simulink model "MON_sl_after_replacement3"  (R2016a)
settings: Solver=FixedStepDiscrete  StartTime=0.0  StopTime=10.0  RelTol=1e-3
undefined symbols (not defined in the file or in its folder): BRAKE_PRESSURE_LO, BRAKE_PRESSURE_MAX, BRAKE_PRESSURE_MED, dt, LO, MANUAL, MAX, MED
libraries: BSCU_lib x3, simulink x1
Description:
  | BSCU Monitor Function Model
settings Model: ModelType=Feature  MBDTemplateVer=1.1  sldv_blockreplacement_configurable_lib=MON_sl_after_rt3_lib  LastModifiedBy=jdbackes
settings DataIOCC: LimitDataPoints=on
settings DebuggingCC: ArtificialAlgebraicLoopMsg=none  AllowSymbolicDim=off
settings ModelReferenceCC: PropagateSignalLabelsOutOfModel=off
settings RTWCC: Description=Generic Real-Time Target
settings GRTTargetCC: GeneratePreprocessorConditionals=Use local settings
settings ConfigComp: DVMode=PropertyProving  DVTestSuiteOptimization=CombinedObjectives (Nonlinear Extended)  DVAssertions=EnableAll  DVProofAssumptions=EnableAll  DVDisplayReport=off

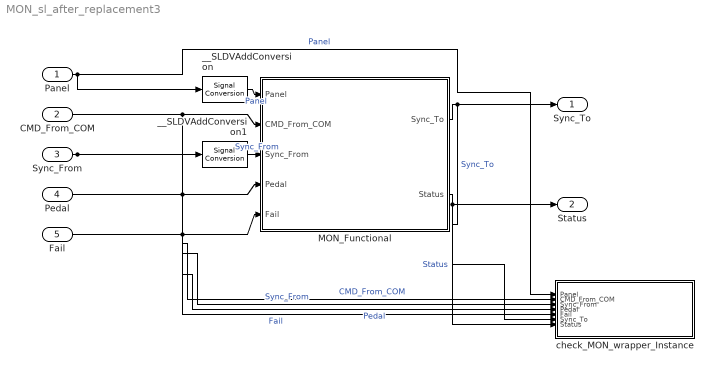
== system MON_sl_after_replacement3 ==
  Panel : Inport  OutDataTypeStr=Bus: PanelMsgImpl  SampleTime=dt  Interpolate=off  BusOutputAsStruct=on
  CMD_From_COM : Inport  Port=2  OutDataTypeStr=int32  SampleTime=dt  Interpolate=off
  Sync_From : Inport  Port=3  OutDataTypeStr=Bus: SyncMsgImpl  SampleTime=dt  Interpolate=off  BusOutputAsStruct=on
  Pedal : Inport  Port=4  OutDataTypeStr=int32  SampleTime=dt  Interpolate=off
  Fail : Inport  Port=5  OutDataTypeStr=boolean  SampleTime=dt  Interpolate=off
  MON_Functional : Subsystem  TreatAsAtomicUnit=on  mask(Sldv ModelReference(Model name:MON_Functional) Replacement){ModelName=MON_Functional, ParameterArgumentNames=, ParameterArgumentValues=, SimulationMode=Normal}
      mask help: Replacement for the Model Reference block that references the model MON_Functional. If Model arguments are specified on the Model Reference block, then they will appear in the mask parameters.
  __SLDVAddConversion : SignalConversion  ConversionOutput=Virtual bus  OverrideOpt=off
  __SLDVAddConversion1 : SignalConversion  ConversionOutput=Virtual bus  OverrideOpt=off
  check_MON_wrapper_Instance : MATLAB Function  TreatAsAtomicUnit=on  mask(VerificationSubsystem){}
  Sync_To : Outport  OutDataTypeStr=Bus: SyncMsgImpl  BusOutputAsStruct=on
  Status : Outport  Port=2  OutDataTypeStr=Bus: ChannelStatusImpl  BusOutputAsStruct=on
  wires:
  MON_Functional/1(Sync_To) -> Sync_To/1, check_MON_wrapper_Instance/6(Sync_To)  "Sync_To"
  MON_Functional/2(Status) -> Status/1, check_MON_wrapper_Instance/7(Status)  "Status"
  Panel/1 -> check_MON_wrapper_Instance/1(Panel), __SLDVAddConversion/1  "Panel"
  CMD_From_COM/1 -> MON_Functional/2(CMD_From_COM), check_MON_wrapper_Instance/2(CMD_From_COM)  "CMD_From_COM"
  Sync_From/1 -> check_MON_wrapper_Instance/3(Sync_From), __SLDVAddConversion1/1  "Sync_From"
  Pedal/1 -> MON_Functional/4(Pedal), check_MON_wrapper_Instance/4(Pedal)  "Pedal"
  Fail/1 -> MON_Functional/5(Fail), check_MON_wrapper_Instance/5(Fail)  "Fail"
  __SLDVAddConversion/1 -> MON_Functional/1(Panel)  "Panel"
  __SLDVAddConversion1/1 -> MON_Functional/3(Sync_From)  "Sync_From"

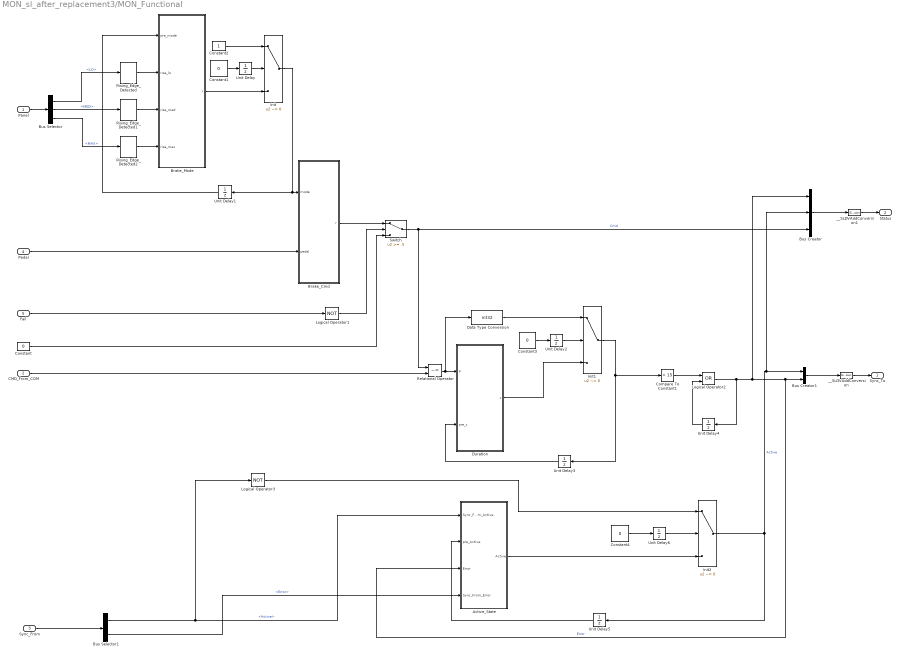
== system MON_sl_after_replacement3/MON_Functional ==
  Panel : Inport  OutDataTypeStr=Bus: PanelMsgImpl  SampleTime=[0.01,0]
  CMD_From_COM : Inport  Port=2  OutDataTypeStr=int32  PortDimensions=1  SampleTime=[0.01,0]
  Sync_From : Inport  Port=3  OutDataTypeStr=Bus: SyncMsgImpl  SampleTime=[0.01,0]
  Pedal : Inport  Port=4  OutDataTypeStr=int32  PortDimensions=1  SampleTime=[0.01,0]
  Fail : Inport  Port=5  OutDataTypeStr=boolean  PortDimensions=1  SampleTime=[0.01,0]
  Active_State : Stateflow chart  TreatAsAtomicUnit=on
  Brake_Cmd : Stateflow chart  TreatAsAtomicUnit=on
  Brake_Mode : Stateflow chart  TreatAsAtomicUnit=on
  Bus Creator : BusCreator  Inputs='Error','Active','Cmd'  OutDataTypeStr=Bus: ChannelStatusImpl  NonVirtualBus=on
  Bus Creator1 : BusCreator  Inputs='Active','Error'  OutDataTypeStr=Bus: SyncMsgImpl  NonVirtualBus=on
  Bus Selector : BusSelector  OutputSignals=LO,MED,MAX
  Bus Selector1 : BusSelector  OutputSignals=Active,Error
  Compare To Constant1 : simulink/Logic and Bit Operations/Compare To Constant  relop=>  const=15  OutDataTypeStr=boolean
  Constant : Constant  Value=0  OutDataTypeStr=int32
  Constant1 : Constant  DisableCoverage=on  Value=0  OutDataTypeStr=boolean
  Constant2 : Constant  OutDataTypeStr=int32
  Constant3 : Constant  DisableCoverage=on  Value=0  OutDataTypeStr=boolean
  Constant4 : Constant  DisableCoverage=on  Value=0  OutDataTypeStr=boolean
  Data Type Conversion : DataTypeConversion  OutDataTypeStr=int32
  Duration : Stateflow chart  TreatAsAtomicUnit=on
  Init : Switch  Criteria=u2 ~= 0  OutDataTypeStr=Inherit: Inherit via back propagation  ZeroCross=off  InputSameDT=on
  Init1 : Switch  Criteria=u2 ~= 0  OutDataTypeStr=Inherit: Inherit via back propagation  ZeroCross=off  InputSameDT=on
  Init2 : Switch  Criteria=u2 ~= 0  OutDataTypeStr=Inherit: Inherit via back propagation  ZeroCross=off  InputSameDT=on
  Logical Operator1 : Logic  Operator=NOT  OutDataTypeStr=boolean
  Logical Operator2 : Logic  Operator=OR  OutDataTypeStr=boolean
  Logical Operator3 : Logic  Operator=NOT  OutDataTypeStr=boolean
  Relational Operator : RelationalOperator  Operator=~=  OutDataTypeStr=boolean  ZeroCross=off  InputSameDT=on
  Rising_Edge_Detected : BSCU_lib/Rising_Edge_Detected
  Rising_Edge_Detected1 : BSCU_lib/Rising_Edge_Detected
  Rising_Edge_Detected2 : BSCU_lib/Rising_Edge_Detected
  Switch : Switch  Description=May be used within well defined functions, or functions that soley define logical expressions.  Threshold=.5  ZeroCross=off  InputSameDT=on
  Unit Delay{,1..2,6} (4 alike) : UnitDelay  InitialCondition=1  SampleTime=-1
      settings: AttributesFormatString=<Init = %<InitialCondition>>
  Unit Delay3 : UnitDelay  SampleTime=-1
      settings: AttributesFormatString=<Init = %<InitialCondition>>
  Unit Delay4 : UnitDelay  SampleTime=-1
      settings: AttributesFormatString=<Init = %<InitialCondition>>
  Unit Delay5 : UnitDelay  SampleTime=-1
      settings: AttributesFormatString=<Init = %<InitialCondition>>
  __SLDVAddConversion : SignalConversion  ConversionOutput=Virtual bus  OverrideOpt=off
  __SLDVAddConversion1 : SignalConversion  ConversionOutput=Virtual bus  OverrideOpt=off
  Sync_To : Outport  OutDataTypeStr=Bus: SyncMsgImpl
  Status : Outport  Port=2  OutDataTypeStr=Bus: ChannelStatusImpl
  wires:
  Unit Delay6/1 -> Init2/2
  Unit Delay5/1 -> Active_State/2(pre_Active)
  Unit Delay4/1 -> Logical Operator2/2
  Unit Delay3/1 -> Duration/2(pre_c)
  Unit Delay1/1 -> Brake_Mode/1(pre_mode)
  Init2/1 -> Unit Delay5/1, Bus Creator/2, Bus Creator1/1  "Active"
  Logical Operator3/1 -> Init2/1
  Constant4/1 -> Unit Delay6/1
  Active_State/1(Active) -> Init2/3
  Init1/1 -> Compare To Constant1/1, Unit Delay3/1
  Data Type Conversion/1 -> Init1/1
  Constant3/1 -> Unit Delay2/1
  Unit Delay2/1 -> Init1/2
  Duration/1(c) -> Init1/3
  Constant2/1 -> Init/1
  Constant1/1 -> Unit Delay/1
  Unit Delay/1 -> Init/2
  Bus Selector1/2 -> Active_State/4(Sync_From_Error)  "<Error>"
  Bus Selector1/1 -> Logical Operator3/1, Active_State/1(Sync_From_Active)  "<Active>"
  Sync_From/1 -> Bus Selector1/1
  Compare To Constant1/1 -> Logical Operator2/1
  Logical Operator2/1 -> Unit Delay4/1, Bus Creator/1, Active_State/3(Error), Bus Creator1/2  "Error"
  Relational Operator/1 -> Data Type Conversion/1, Duration/1(p)
  CMD_From_COM/1 -> Relational Operator/2
  Constant/1 -> Switch/3
  Switch/1 -> Bus Creator/3, Relational Operator/1  "Cmd"
  Logical Operator1/1 -> Switch/2
  Brake_Cmd/1(r) -> Switch/1
  Fail/1 -> Logical Operator1/1
  Pedal/1 -> Brake_Cmd/2(pedal)
  Rising_Edge_Detected2/1 -> Brake_Mode/4(rise_max)
  Rising_Edge_Detected1/1 -> Brake_Mode/3(rise_med)
  Rising_Edge_Detected/1 -> Brake_Mode/2(rise_lo)
  Bus Selector/3 -> Rising_Edge_Detected2/1  "<MAX>"
  Bus Selector/2 -> Rising_Edge_Detected1/1  "<MED>"
  Bus Selector/1 -> Rising_Edge_Detected/1  "<LO>"
  Panel/1 -> Bus Selector/1
  Init/1 -> Unit Delay1/1, Brake_Cmd/1(mode)
  Brake_Mode/1(r) -> Init/3
  Bus Creator1/1 -> __SLDVAddConversion/1
  __SLDVAddConversion/1 -> Sync_To/1
  Bus Creator/1 -> __SLDVAddConversion1/1
  __SLDVAddConversion1/1 -> Status/1

== stateflow chart MON_sl_after_replacement3/MON_Functional/Brake_Cmd ==
  (default) -> (junction 4789)
  (junction 4789) -> (junction 4790) [order 1] : [mode == LO]
  (junction 4789) -> (junction 4791) [order 2]
  (junction 4790) -> (junction 4798) : {
      | r = BRAKE_PRESSURE_LO;
      | }
  (junction 4791) -> (junction 4792) [order 1] : [mode == MED ]
  (junction 4791) -> (junction 4793) [order 2]
  (junction 4792) -> (junction 4797) : {
      | r = BRAKE_PRESSURE_MED;
      | }
  (junction 4793) -> (junction 4794) [order 1] : [mode == MAX]
  (junction 4793) -> (junction 4800) [order 2]
  (junction 4794) -> (junction 4796) : {
      | r = BRAKE_PRESSURE_MAX;
      | }
  (junction 4800) -> (junction 4795) : {
      | r = pedal;
      | }
  (junction 4796) -> (junction 4795)
  (junction 4797) -> (junction 4796)
  (junction 4798) -> (junction 4797)
  (junction 4795) -> (junction 4799)
  data: mode input int32; pedal input int32; r output int32; MANUAL parameter =1; LO parameter =2; MED parameter =3; MAX parameter =4; BRAKE_PRESSURE_LO parameter; BRAKE_PRESSURE_MAX parameter; BRAKE_PRESSURE_MED parameter

== matlab function MON_sl_after_replacement3/check_MON_wrapper_Instance ==
  data: Panel input; CMD_From_COM input; Sync_From input; Pedal input; Fail input; Sync_To input; Status input
function check_MON_wrapper_Instance(Panel, CMD_From_COM, Sync_From, Pedal, Fail, Sync_To, Status)

persistent pre_c_Agree_Nodes__Duration_0
persistent pre_p_Agree_Nodes__Rise_2_Agree_Nodes__Brake_Mode_0
persistent pre_mode_Agree_Nodes__Brake_Mode_0
persistent pre_Active
persistent first_time
persistent pre_p_Agree_Nodes__Rise_0_Agree_Nodes__Brake_Mode_0
persistent pre_p_Agree_Nodes__Rise_1_Agree_Nodes__Brake_Mode_0
persistent pre_r_Agree_Nodes__Latch_0

Primary_Side = false;
max_Agree_Nodes__Brake_Mode_0 = Panel.MAX;
p_Agree_Nodes__Rise_2_Agree_Nodes__Brake_Mode_0 = max_Agree_Nodes__Brake_Mode_0;

if isempty(pre_p_Agree_Nodes__Rise_2_Agree_Nodes__Brake_Mode_0)
	pre_p_Agree_Nodes__Rise_2_Agree_Nodes__Brake_Mode_0 = (false);
end


if isempty(first_time)
	first_time = true;
end

r_Agree_Nodes__Rise_2_Agree_Nodes__Brake_Mode_0 = arrowFunction(first_time,false, (not(pre_p_Agree_Nodes__Rise_2_Agree_Nodes__Brake_Mode_0) && p_Agree_Nodes__Rise_2_Agree_Nodes__Brake_Mode_0));
lo_Agree_Nodes__Brake_Mode_0 = Panel.LO;
p_Agree_Nodes__Rise_0_Agree_Nodes__Brake_Mode_0 = lo_Agree_Nodes__Brake_Mode_0;

if isempty(pre_p_Agree_Nodes__Rise_0_Agree_Nodes__Brake_Mode_0)
	pre_p_Agree_Nodes__Rise_0_Agree_Nodes__Brake_Mode_0 = (false);
end

r_Agree_Nodes__Rise_0_Agree_Nodes__Brake_Mode_0 = arrowFunction(first_time,false, (not(pre_p_Agree_Nodes__Rise_0_Agree_Nodes__Brake_Mode_0) && p_Agree_Nodes__Rise_0_Agree_Nodes__Brake_Mode_0));
med_Agree_Nodes__Brake_Mode_0 = Panel.MED;
p_Agree_Nodes__Rise_1_Agree_Nodes__Brake_Mode_0 = med_Agree_Nodes__Brake_Mode_0;

if isempty(pre_p_Agree_Nodes__Rise_1_Agree_Nodes__Brake_Mode_0)
	pre_p_Agree_Nodes__Rise_1_Agree_Nodes__Brake_Mode_0 = (false);
end

r_Agree_Nodes__Rise_1_Agree_Nodes__Brake_Mode_0 = arrowFunction(first_time,false, (not(pre_p_Agree_Nodes__Rise_1_Agree_Nodes__Brake_Mode_0) && p_Agree_Nodes__Rise_1_Agree_Nodes__Brake_Mode_0));

if isempty(pre_mode_Agree_Nodes__Brake_Mode_0)
	pre_mode_Agree_Nodes__Brake_Mode_0 = int32(0);
end

r_Agree_Nodes__Brake_Mode_0 = arrowFunction(first_time,int32(1), ifFunction((isequal(pre_mode_Agree_Nodes__Brake_Mode_0, int32(2)) && r_Agree_Nodes__Rise_0_Agree_Nodes__Brake_Mode_0), int32(1), ifFunction((isequal(pre_mode_Agree_Nodes__Brake_Mode_0, int32(3)) && r_Agree_Nodes__Rise_1_Agree_Nodes__Brake_Mode_0), int32(1), ifFunction((isequal(pre_mode_Agree_Nodes__Brake_Mode_0, int32(4)) && r_Agree_Nodes__Rise_2_Agree_Nodes__Brake_Mode_0), int32(1), ifFunction(((pre_mode_Agree_Nodes__Brake_Mode_0 ~= int32(2)) && r_Agree_Nodes__Rise_0_Agree_Nodes__Brake_Mode_0), int32(2), ifFunction(((pre_mode_Agree_Nodes__Brake_Mode_0 ~= int32(3)) && r_Agree_Nodes__Rise_1_Agree_Nodes__Brake_Mode_0), int32(3), ifFunction(((pre_mode_Agree_Nodes__Brake_Mode_0 ~= int32(4)) && r_Agree_Nodes__Rise_2_Agree_Nodes__Brake_Mode_0), int32(4), pre_mode_Agree_Nodes__Brake_Mode_0)))))));
Mode = r_Agree_Nodes__Brake_Mode_0;
p_Agree_Nodes__Duration_0 = not(isequal(Status.Cmd, CMD_From_COM));
b_Agree_Nodes__b2i_0_Agree_Nodes__Duration_0 = p_Agree_Nodes__Duration_0;
i_Agree_Nodes__b2i_0_Agree_Nodes__Duration_0 = ifFunction(b_Agree_Nodes__b2i_0_Agree_Nodes__Duration_0, int32(1), int32(0));

if isempty(pre_c_Agree_Nodes__Duration_0)
	pre_c_Agree_Nodes__Duration_0 = int32(0);
end

c_Agree_Nodes__Duration_0 = arrowFunction(first_time,i_Agree_Nodes__b2i_0_Agree_Nodes__Duration_0, ifFunction(p_Agree_Nodes__Duration_0, (pre_c_Agree_Nodes__Duration_0 + int32(1)), int32(0)));
p_Agree_Nodes__Latch_0 = (c_Agree_Nodes__Duration_0 > int32(15));

if isempty(pre_r_Agree_Nodes__Latch_0)
	pre_r_Agree_Nodes__Latch_0 = (false);
end

r_Agree_Nodes__Latch_0 = arrowFunction(first_time,p_Agree_Nodes__Latch_0, (p_Agree_Nodes__Latch_0 || pre_r_Agree_Nodes__Latch_0));
Error = r_Agree_Nodes__Latch_0;

if isempty(pre_Active)
	pre_Active = (false);
end

Active = arrowFunction(first_time,not(Sync_From.Active), ifFunction(Error, false, ifFunction((((pre_Active && Sync_From.Active) && not(Sync_From.Error)) && not(Primary_Side)), false, ifFunction((not(pre_Active) && (not(Sync_From.Active) || Sync_From.Error)), true, pre_Active))));
pedal_Agree_Nodes__Brake_Cmd_0 = Pedal;
mode_Agree_Nodes__Brake_Cmd_0 = Mode;
r_Agree_Nodes__Brake_Cmd_0 = ifFunction(isequal(mode_Agree_Nodes__Brake_Cmd_0, int32(2)), int32(170), ifFunction(isequal(mode_Agree_Nodes__Brake_Cmd_0, int32(3)), int32(340), ifFunction(isequal(mode_Agree_Nodes__Brake_Cmd_0, int32(4)), int32(510), pedal_Agree_Nodes__Brake_Cmd_0)));
GUARANTEE0 = impliesFunction(not(Fail), isequal(Status.Cmd, r_Agree_Nodes__Brake_Cmd_0));
GUARANTEE1 = ~isequal(Status.Error, Error);
GUARANTEE2 = isequal(Sync_To.Error, Error);
GUARANTEE3 = isequal(Status.Active, Active);
GUARANTEE4 = isequal(Sync_To.Active, Active);
mode_Agree_Nodes__Brake_Mode_0 = Mode;
nodeLemma0_Agree_Nodes__Duration_0 = (c_Agree_Nodes__Duration_0 >= int32(0));
pre_c_Agree_Nodes__Duration_0 = c_Agree_Nodes__Duration_0;
pre_p_Agree_Nodes__Rise_2_Agree_Nodes__Brake_Mode_0 = p_Agree_Nodes__Rise_2_Agree_Nodes__Brake_Mode_0;
pre_mode_Agree_Nodes__Brake_Mode_0 = mode_Agree_Nodes__Brake_Mode_0;
pre_Active = Active;
first_time = false;
pre_p_Agree_Nodes__Rise_0_Agree_Nodes__Brake_Mode_0 = p_Agree_Nodes__Rise_0_Agree_Nodes__Brake_Mode_0;
pre_p_Agree_Nodes__Rise_1_Agree_Nodes__Brake_Mode_0 = p_Agree_Nodes__Rise_1_Agree_Nodes__Brake_Mode_0;
pre_r_Agree_Nodes__Latch_0 = r_Agree_Nodes__Latch_0;

sldv.prove(GUARANTEE0)

sldv.prove(GUARANTEE1)

sldv.prove(GUARANTEE2)

sldv.prove(GUARANTEE3)

sldv.prove(GUARANTEE4)

sldv.prove(nodeLemma0_Agree_Nodes__Duration_0)

end

function output = ifFunction(cond, ifBranch, elseBranch)
if (cond)
	output = ifBranch;
else
	output = elseBranch;
end
end

function output = arrowFunction(first_time, left, right)
if (first_time)
	output = left;
else
	output = right;
end
end

function output = impliesFunction(left, right)
	output = (not(left) || right);
end

== stateflow chart MON_sl_after_replacement3/MON_Functional/Brake_Mode ==
  (default) -> (junction 4789)
  (junction 4789) -> (junction 4790) [order 1] : [  ((pre_mode == LO) && rise_lo) || ...
      |    ((pre_mode == MED) && rise_med) || ...
      |    ((pre_mode == MAX) && rise_max)
      | ]
  (junction 4789) -> (junction 4791) [order 2]
  (junction 4790) -> (junction 4798) : {
      | r = MANUAL;
      | }
  (junction 4791) -> (junction 4792) [order 1] : [  (pre_mode != LO) && rise_lo ]
  (junction 4791) -> (junction 4793) [order 2]
  (junction 4792) -> (junction 4797) : {
      | r = LO;
      | }
  (junction 4793) -> (junction 4794) [order 1] : [ (pre_mode != MED) && rise_med ]
  (junction 4793) -> (junction 4800) [order 2]
  (junction 4794) -> (junction 4796) : {
      | r = MED;
      | }
  (junction 4800) -> (junction 4808) [order 1] : [ (pre_mode != MAX) && rise_max ]
  (junction 4800) -> (junction 4795) [order 2] : {
      | r = pre_mode;
      | }
  (junction 4808) -> (junction 4810) : {
      | r = MAX;
      | }
  (junction 4810) -> (junction 4795)
  (junction 4796) -> (junction 4810)
  (junction 4797) -> (junction 4796)
  (junction 4798) -> (junction 4797)
  (junction 4795) -> (junction 4799)
  data: pre_mode input int32; rise_lo input boolean; rise_med input boolean; rise_max input boolean; r output int32; MANUAL parameter =1; LO parameter =2; MED parameter =3; MAX parameter =4

== stateflow chart MON_sl_after_replacement3/MON_Functional/Active_State ==
  (default) -> (junction 4848)
  (junction 4848) -> (junction 4849) [order 1] : [Error]
  (junction 4848) -> (junction 4850) [order 2]
  (junction 4849) -> (junction 4857) : {Active = false;}
  (junction 4850) -> (junction 4851) [order 1] : [pre_Active && Sync_From_Active && (! Sync_From_Error) && (! Primary_Side) ]
  (junction 4850) -> (junction 4852) [order 2]
  (junction 4851) -> (junction 4856) : {Active = false;}
  (junction 4852) -> (junction 4853) [order 1] : [(!pre_Active) && ( (!Sync_From_Active) || Sync_From_Error)]
  (junction 4852) -> (junction 4854) [order 2] : {Active = pre_Active;}
  (junction 4853) -> (junction 4855) : {Active = true;}
  (junction 4855) -> (junction 4854)
  (junction 4856) -> (junction 4855)
  (junction 4857) -> (junction 4856)
  (junction 4854) -> (junction 4858)
  data: Sync_From_Active input boolean; Active output boolean; pre_Active input boolean; Error input boolean; Sync_From_Error input boolean; Primary_Side parameter

== stateflow chart MON_sl_after_replacement3/MON_Functional/Duration ==
  (default) -> (junction 4827)
  (junction 4827) -> (junction 4828) [order 1] : [p]
  (junction 4827) -> (junction 4829) [order 2] : {c = 0;}
  (junction 4828) -> (junction 4830) : {c = pre_c+1;}
  (junction 4830) -> (junction 4829)
  (junction 4829) -> (junction 4831)
  data: p input boolean; c output int32; pre_c input int32
